simulink model "GUIADO1"  (R2021b)
settings: Solver=VariableStepAuto  StartTime=0.0  StopTime=10.0  RelTol=1e-3
values from neighbouring files (symbols this model uses):
  fp = [t1;t2;t3]    [creacionestructurasborrador.m]    (also in flight_plan.m = [sid,wps,iap]; flight_plan_eval.m = [t1;tabla2;t3]; flight_plan_old.m = [sid,wps,iap]; flight_plan_struct.m = [t1;tabla2;t3])
libraries: simulink x4
settings Model: Creator=patri  LastModifiedBy=verti

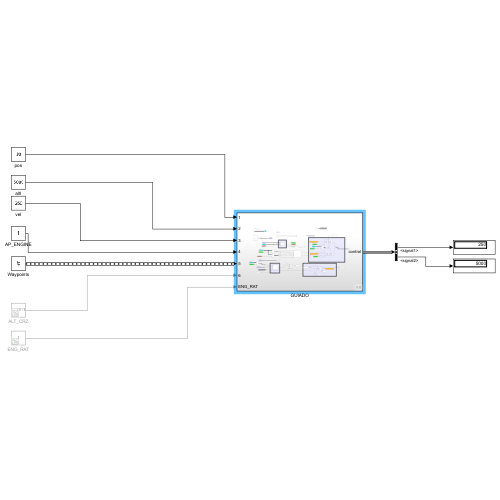
[thumbnail: Simulink's stored preview of the top-level diagram]
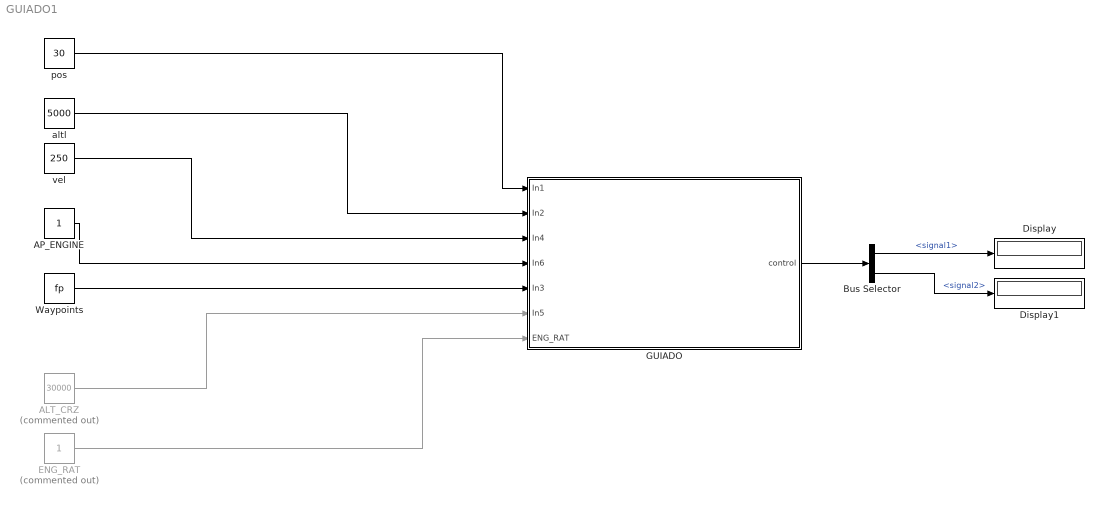
== system GUIADO1 ==
  ALT_CRZ : Constant  Commented=on  Value=30000
  AP_ENGINE : Constant
  Bus Selector : BusSelector  OutputSignals=signal1,signal2
  Display : Display
  Display1 : Display
  ENG_RAT : Constant  Commented=on
  GUIADO : Subsystem
  Waypoints : Constant  RequirementInfo={} %GIDa_b85dfdf9_dbd9_42fc_8c21_ccd8d1c0f83a  Value=fp  OutDataTypeStr=Bus: BUS_FP
  altl : Constant  RequirementInfo={} %GIDa_24b8d891_c115_477c_8ce2_324cbd10ab9b  Value=5000
  pos : Constant  RequirementInfo={} %GIDa_e0c8f14f_9d58_42a1_8d51_6b8f44cf598c  Value=30
  vel : Constant  RequirementInfo={} %GIDa_4ea119f1_ae62_469e_9a59_9854960f9910  Value=250
  wires:
  altl/1 -> GUIADO/2(In2)
  pos/1 -> GUIADO/1(In1)
  vel/1 -> GUIADO/3(In4)
  Waypoints/1 -> GUIADO/5(In3)
  ENG_RAT/1 -> GUIADO/7(ENG_RAT)
  ALT_CRZ/1 -> GUIADO/6(In5)
  AP_ENGINE/1 -> GUIADO/4(In6)
  GUIADO/1(control) -> Bus Selector/1
  Bus Selector/2 -> Display1/1  "<signal2>"
  Bus Selector/1 -> Display/1  "<signal1>"

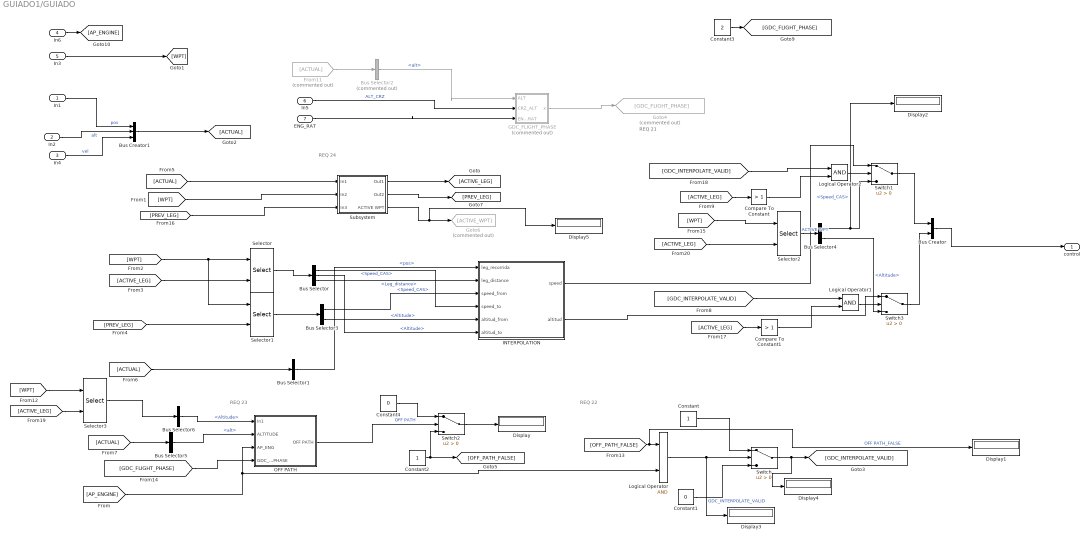
== system GUIADO1/GUIADO ==
  note: REQ 24
  note: REQ 21
  note: REQ 22
  note: REQ 23
  In1 : Inport  RequirementInfo={} %GIDa_c953edaa_2252_4c9d_8426_3d6d548ae88e
  In2 : Inport  RequirementInfo={} %GIDa_547d8447_87e3_4c66_b2f0_2f18738a3143  Port=2
  In4 : Inport  Port=3
  In6 : Inport  Port=4
  In3 : Inport  Port=5
  In5 : Inport  Port=6
  ENG_RAT : Inport  Port=7
  Bus Creator : BusCreator  RequirementInfo={} %GIDa_01f04d6e_35c0_4dde_ad67_30f95352da07  Inputs=2
  Bus Creator1 : BusCreator  RequirementInfo={} %GIDa_002cc265_eead_4a65_9c30_5969614079fc  Inputs=3
  Bus Selector : BusSelector  RequirementInfo={} %GIDa_c4a2b3b9_26f5_4370_8f3c_fb220d56f2b1  OutputSignals=Speed_CAS,Altitude,Leg_distance
  Bus Selector1 : BusSelector  RequirementInfo={} %GIDa_f06f846a_f20a_4ebb_91a5_5d7a160146ce  OutputSignals=pos
  Bus Selector2 : BusSelector  RequirementInfo={} %GIDa_67f18f8f_3d6a_4122_98a0_2b1872e91802  Commented=on  OutputSignals=alt
  Bus Selector3 : BusSelector  RequirementInfo={} %GIDa_3179e8d2_440f_49e3_a760_530bcd082419  OutputSignals=Speed_CAS,Altitude
  Bus Selector4 : BusSelector  OutputSignals=Speed_CAS,Altitude
  Bus Selector5 : BusSelector  OutputSignals=alt
  Bus Selector6 : BusSelector  RequirementInfo={} %GIDa_8bc3223d_0b7f_40fb_a6f5_c44549fe0063  OutputSignals=Altitude
  Compare To Constant : simulink/Logic and Bit Operations/Compare To Constant  relop=>  const=1  OutDataTypeStr=boolean
  Compare To Constant1 : simulink/Logic and Bit Operations/Compare To Constant  relop=>  const=1  OutDataTypeStr=boolean
  Constant : Constant  RequirementInfo={} %GIDa_2498b4de_2ac4_48bd_8c57_f50d97e9c0ba
  Constant1 : Constant  RequirementInfo={} %GIDa_d7690ee0_1221_4b71_bf56_b8fc32b8c303  Value=0
  Constant2 : Constant  RequirementInfo={} %GIDa_5ab9040d_ce11_44b0_aa60_fbd51e1cd284
  Constant3 : Constant  Value=2
  Constant4 : Constant  Value=0
  Display{,1..5} (6 alike) : Display
      Display settings: RequirementInfo={} %GIDa_70cf4f96_cbbf_4ac9_a295_881ac1100427
  From11 : From  RequirementInfo={} %GIDa_ba6d5a2b_274e_4e09_a48e_951a476e8210  Commented=on  GotoTag=ACTUAL
  GDC_FLIGHT_PHASE : Stateflow chart  RequirementInfo={} %GIDa_738fd6ca_d950_41b5_85a8_34e3c94ad36e  Commented=on  TreatAsAtomicUnit=on
  Goto4 : Goto  RequirementInfo={} %GIDa_7a49e31f_81d1_4690_999b_ac34b1e525ce  Commented=on  GotoTag=GDC_FLIGHT_PHASE
  Goto6 : Goto  RequirementInfo={} %GIDa_8f7bf202_a020_4678_839c_04c19c1a886f  Commented=on  GotoTag=ACTIVE_WPT
  INTERPOLATION : MATLAB Function  RequirementInfo={} %GIDa_d69dad2e_6c63_4369_b768_ec321f42f021  TreatAsAtomicUnit=on
  Logical Operator : Logic  RequirementInfo={} %GIDa_5b6a2d32_a21a_44cf_8e21_c6f9ba66fa3f  AllPortsSameDT=off  OutDataTypeStr=boolean
  Logical Operator1 : Logic  RequirementInfo={} %GIDa_0c25b4f0_cec9_4cfd_a32d_1709ca197c58  AllPortsSameDT=off  OutDataTypeStr=boolean
  Logical Operator2 : Logic  RequirementInfo={} %GIDa_21f84cc6_6a89_4154_be44_27295376b10c  AllPortsSameDT=off  OutDataTypeStr=boolean
  OFF PATH : Subsystem  RequirementInfo={} %GIDa_fce4e217_4c17_48f9_b389_237c9766bcea
  Selector : Selector  RequirementInfo={} %GIDa_aa8aed47_c89b_4cd5_946f_b9cf7f706766  InputPortWidth=12  IndexOptions=Index vector (port)  Indices=[1 3]  OutputSizes=1
  Selector1 : Selector  RequirementInfo={} %GIDa_3f3fe1df_2ad1_4bff_9a1e_105282a61a3c  InputPortWidth=12  IndexOptions=Index vector (port)  Indices=[1 3]  OutputSizes=1
  Selector2 : Selector  RequirementInfo={} %GIDa_63b54d3c_663a_435b_9dc1_1443cfa2f20c  InputPortWidth=12  IndexOptions=Index vector (port)  Indices=[1 3]  OutputSizes=1
  Selector3 : Selector  InputPortWidth=12  IndexOptions=Index vector (port)  Indices=[1 3]  OutputSizes=1
  Subsystem : Subsystem  RequirementInfo={} %GIDa_d93d8f36_c3e8_4324_81a1_465d92c3f292
  Switch : Switch  RequirementInfo={} %GIDa_1e34e9e4_1641_447b_8b9c_841ac2d26e67  Criteria=u2 > Threshold
  Switch1 : Switch  RequirementInfo={} %GIDa_27784f20_4fa4_452b_ae6f_1814d084a7da  Criteria=u2 > Threshold
  Switch2 : Switch  RequirementInfo={} %GIDa_46de363e_4d07_48d3_90c2_fbede5ff2297  Criteria=u2 > Threshold
  Switch3 : Switch  RequirementInfo={} %GIDa_d53d12ca_965a_40d8_8672_d8cd2ef96e8e  Criteria=u2 > Threshold
  control : Outport  RequirementInfo={} %GIDa_4dbd6388_d035_474b_bcb7_a1e098248e58
  wires:
  [ACTUAL] -> Bus Selector5/1
  Bus Selector/1 -> INTERPOLATION/4(speed_to)  "<Speed_CAS>"
  Compare To Constant/1 -> Logical Operator2/2
  Constant1/1 -> Switch/3
  Selector1/1 -> Bus Selector3/1
  Switch/1 -> Display4/1, [GDC_INTERPOLATE_VALID]
  Subsystem/2(Out2) -> [PREV_LEG]
  From11/1 -> Bus Selector2/1
  Switch2/1 -> Display/1
  [GDC_FLIGHT_PHASE] -> OFF PATH/4(GDC_FLIGHT_PHASE)
  [ACTUAL] -> Subsystem/1(In1)
  Bus Selector3/1 -> INTERPOLATION/3(speed_from)  "<Speed_CAS>"
  Bus Selector3/2 -> INTERPOLATION/5(altitud_from)  "<Altitude>"
  In2/1 -> Bus Creator1/2  "alt"
  INTERPOLATION/1(speed) -> Switch1/1
  [ACTIVE_LEG] -> Compare To Constant/1
  Compare To Constant1/1 -> Logical Operator1/2
  Logical Operator2/1 -> Switch1/2
  [ACTIVE_LEG] -> Compare To Constant1/1
  Constant2/1 -> Switch2/3, [OFF_PATH_FALSE]
  Switch3/1 -> Bus Creator/2
  [GDC_INTERPOLATE_VALID] -> Logical Operator2/1
  Logical Operator1/1 -> Switch3/2
  [WPT] -> Subsystem/2(In2)
  In3/1 -> [WPT]
  INTERPOLATION/2(altitud) -> Switch3/1
  Bus Creator/1 -> control/1
  Bus Selector/2 -> INTERPOLATION/6(altitud_to)  "<Altitude>"
  Switch1/1 -> Bus Creator/1
  Bus Selector2/1 -> GDC_FLIGHT_PHASE/1(ALT)  "<alt>"
  Constant/1 -> Switch/1
  Logical Operator/1 -> Display3/1, Switch/2  "GDC_INTERPOLATE_VALID"
  Bus Creator1/1 -> [ACTUAL]
  Selector/1 -> Bus Selector/1
  [AP_ENGINE] -> OFF PATH/3(AP_ENG), Logical Operator/2
  [OFF_PATH_FALSE] -> Display1/1, Logical Operator/1  "OFF PATH_FALSE"
  In1/1 -> Bus Creator1/1  "pos"
  [PREV_LEG] -> Subsystem/3(In3)
  [ACTUAL] -> Bus Selector1/1
  Constant4/1 -> Switch2/1
  GDC_FLIGHT_PHASE/1(x) -> Goto4/1
  [WPT] -> Selector1/1, Selector/1
  Subsystem/1(Out1) -> [ACTIVE_LEG]
  OFF PATH/1(OFF PATH) -> Switch2/2  "OFF PATH"
  [GDC_INTERPOLATE_VALID] -> Logical Operator1/1
  [ACTIVE_LEG] -> Selector/2
  In4/1 -> Bus Creator1/3  "vel"
  [ACTIVE_LEG] -> Selector2/2
  [WPT] -> Selector2/1
  Selector2/1 -> Bus Selector4/1  "ACTIVE WPT"
  Bus Selector4/1 -> Display2/1, Switch1/3  "<Speed_CAS>"
  Bus Selector4/2 -> Switch3/3  "<Altitude>"
  [PREV_LEG] -> Selector1/2
  In5/1 -> GDC_FLIGHT_PHASE/2(CRZ_ALT)  "ALT_CRZ"
  ENG_RAT/1 -> GDC_FLIGHT_PHASE/3(ENG_RAT)
  Constant3/1 -> [GDC_FLIGHT_PHASE]
  Bus Selector5/1 -> OFF PATH/2(ALTITUDE)  "<alt>"
  Bus Selector6/1 -> OFF PATH/1(In1)  "<Altitude>"
  [WPT] -> Selector3/1
  Selector3/1 -> Bus Selector6/1
  [ACTIVE_LEG] -> Selector3/2
  In6/1 -> [AP_ENGINE]
  Bus Selector1/1 -> INTERPOLATION/1(leg_recorrida)  "<pos>"
  Bus Selector/3 -> INTERPOLATION/2(leg_distance)  "<Leg_distance>"
  Subsystem/3(ACTIVE WPT) -> Display5/1, Goto6/1

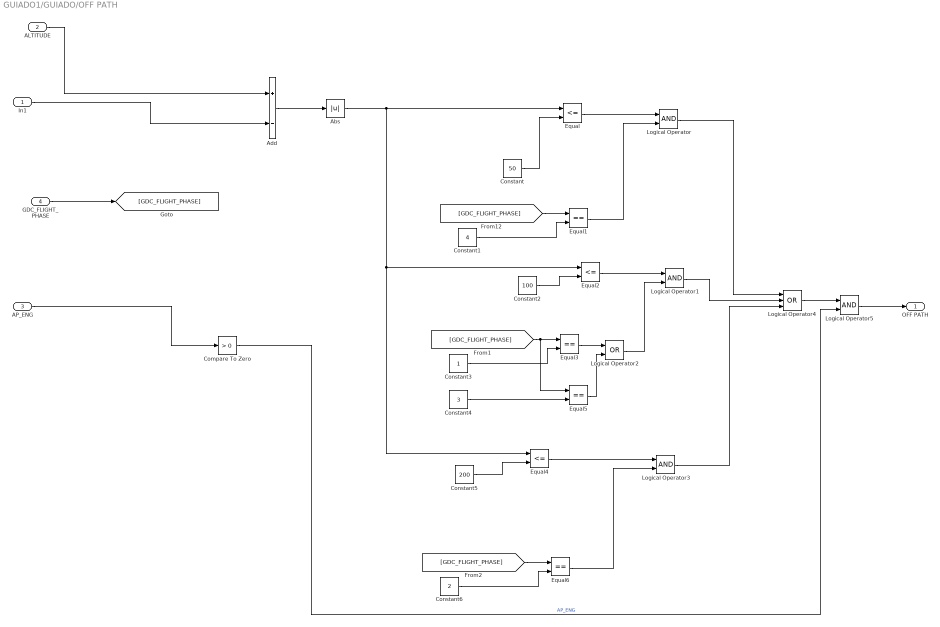
== system GUIADO1/GUIADO/OFF PATH ==
  In1 : Inport  RequirementInfo={} %GIDa_ea188e89_eef4_4315_b4ea_694436859049
  ALTITUDE : Inport  RequirementInfo={} %GIDa_cec92ccd_50af_48ce_99e0_e78f87b5a5dd  Port=2
  AP_ENG : Inport  RequirementInfo={} %GIDa_b5a9fb80_9e70_4b36_a3d4_181a89380a09  Port=3
  GDC_FLIGHT_PHASE : Inport  RequirementInfo={} %GIDa_449a8b27_a283_4b51_85f1_d3db49c09d81  Port=4
  Abs : Abs  RequirementInfo={} %GIDa_db76a9bc_fd40_41b7_b4e9_c8f1fa3f6419
  Add : Sum  RequirementInfo={} %GIDa_1eb463e1_2c0f_4155_9caf_ebd713becfc9  Inputs=+-
  Compare To Zero : simulink/Logic and Bit Operations/Compare To Zero  RequirementInfo={} %GIDa_de6d2e43_5074_4e60_86a5_29e173b01aeb  relop=>  OutDataTypeStr=boolean
  Constant : Constant  RequirementInfo={} %GIDa_50edc1c4_4358_4970_abca_b0e9409f851a  Value=50
  Constant1 : Constant  RequirementInfo={} %GIDa_ee39c8f9_9d82_4b7c_b7b4_7766ecc2abfe  Value=4
  Constant2 : Constant  RequirementInfo={} %GIDa_fa64b539_4baf_4742_984f_2a1e30e52f84  Value=100
  Constant3 : Constant  RequirementInfo={} %GIDa_b30783bd_8107_4173_8871_ce95e60f06e5
  Constant4 : Constant  RequirementInfo={} %GIDa_62456426_7c96_48d7_b64a_6a8d71b153fa  Value=3
  Constant5 : Constant  RequirementInfo={} %GIDa_6ce19b5c_559d_4c88_b743_76247ddbb29b  Value=200
  Constant6 : Constant  RequirementInfo={} %GIDa_176fc83c_97bb_40dd_8d0a_c2bcedeeb068  Value=2
  Equal : RelationalOperator  RequirementInfo={} %GIDa_461bf3d0_5128_4580_83eb_d11cda6f1f54  Operator=<=  OutDataTypeStr=boolean  RndMeth=Simplest
  Equal1 : RelationalOperator  RequirementInfo={} %GIDa_fb95551d_c38f_4b25_a200_648df0e3a261  Operator===  OutDataTypeStr=boolean  RndMeth=Simplest
  Equal2 : RelationalOperator  RequirementInfo={} %GIDa_07670def_aa68_4caa_b5d3_7fed440a0cb2  Operator=<=  OutDataTypeStr=boolean  RndMeth=Simplest
  Equal3 : RelationalOperator  RequirementInfo={} %GIDa_ceb44fc0_0920_4a7b_ba38_e15afd348e9c  Operator===  OutDataTypeStr=boolean  RndMeth=Simplest
  Equal4 : RelationalOperator  RequirementInfo={} %GIDa_b1d64c76_31ce_47f0_b5ac_a43420f1547c  Operator=<=  OutDataTypeStr=boolean  RndMeth=Simplest
  Equal5 : RelationalOperator  RequirementInfo={} %GIDa_2958bcab_fb85_461e_97e2_a6dac5bfcaec  Operator===  OutDataTypeStr=boolean  RndMeth=Simplest
  Equal6 : RelationalOperator  RequirementInfo={} %GIDa_58d89293_8496_455d_9e80_32ec11f8f5c1  Operator===  OutDataTypeStr=boolean  RndMeth=Simplest
  Logical Operator : Logic  RequirementInfo={} %GIDa_cea7d4b5_5f50_4197_98d6_c45754679a30  AllPortsSameDT=off  OutDataTypeStr=boolean
  Logical Operator1 : Logic  RequirementInfo={} %GIDa_f384c015_dcc1_4c97_bf18_ececb565dac7  AllPortsSameDT=off  OutDataTypeStr=boolean
  Logical Operator2 : Logic  RequirementInfo={} %GIDa_d6ad186f_4603_4263_8868_992f6354fea7  Operator=OR  AllPortsSameDT=off  OutDataTypeStr=boolean
  Logical Operator3 : Logic  RequirementInfo={} %GIDa_7655793f_75d5_490d_973e_06ad41c3d157  AllPortsSameDT=off  OutDataTypeStr=boolean
  Logical Operator4 : Logic  RequirementInfo={} %GIDa_9854a055_86ef_4427_9c40_3c0f9a0ce9c4  Operator=OR  Inputs=3  AllPortsSameDT=off  OutDataTypeStr=boolean
  Logical Operator5 : Logic  RequirementInfo={} %GIDa_f127f70b_32ec_43f5_ae91_9e69a0f60159  AllPortsSameDT=off  OutDataTypeStr=boolean
  OFF PATH : Outport  RequirementInfo={} %GIDa_2c7fbac8_b281_4014_84d4_14cf9235134e
  wires:
  AP_ENG/1 -> Compare To Zero/1
  Compare To Zero/1 -> Logical Operator5/2  "AP_ENG"
  ALTITUDE/1 -> Add/1
  Add/1 -> Abs/1
  Constant/1 -> Equal/2
  Abs/1 -> Equal4/1, Equal2/1, Equal/1
  [GDC_FLIGHT_PHASE] -> Equal1/1
  Constant1/1 -> Equal1/2
  Equal1/1 -> Logical Operator/2
  Equal/1 -> Logical Operator/1
  Constant2/1 -> Equal2/2
  Constant3/1 -> Equal3/2
  [GDC_FLIGHT_PHASE] -> Equal5/1, Equal3/1
  Equal2/1 -> Logical Operator1/1
  Equal3/1 -> Logical Operator2/1
  Constant4/1 -> Equal5/2
  Equal5/1 -> Logical Operator2/2
  Logical Operator2/1 -> Logical Operator1/2
  Constant5/1 -> Equal4/2
  Constant6/1 -> Equal6/2
  [GDC_FLIGHT_PHASE] -> Equal6/1
  Equal6/1 -> Logical Operator3/2
  Equal4/1 -> Logical Operator3/1
  Logical Operator/1 -> Logical Operator4/1
  Logical Operator1/1 -> Logical Operator4/2
  Logical Operator3/1 -> Logical Operator4/3
  Logical Operator4/1 -> Logical Operator5/1
  In1/1 -> Add/2
  Logical Operator5/1 -> OFF PATH/1
  GDC_FLIGHT_PHASE/1 -> [GDC_FLIGHT_PHASE]

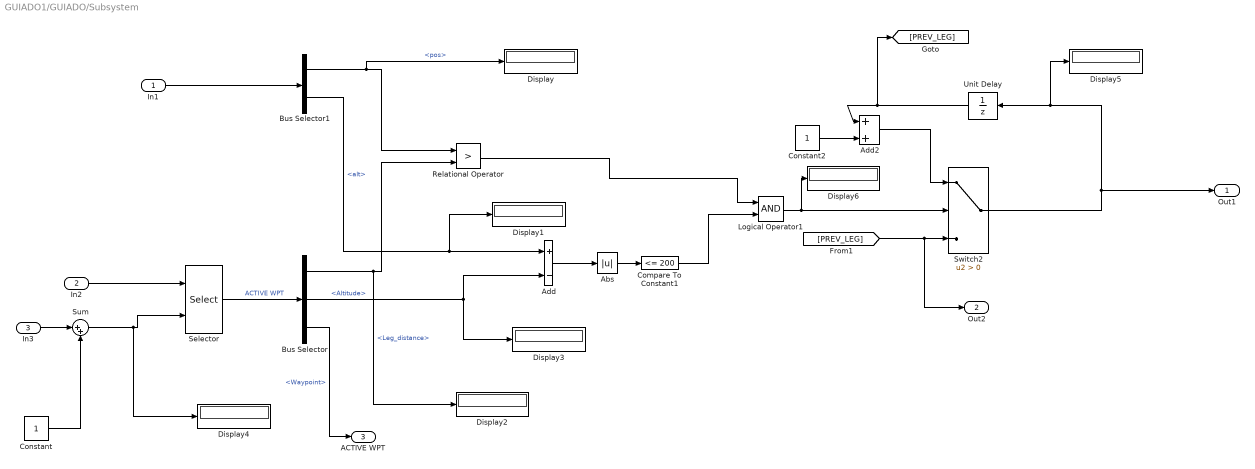
== system GUIADO1/GUIADO/Subsystem ==
  In1 : Inport  RequirementInfo={} %GIDa_0131d32b_efee_4ea4_ac79_6c0467cb0f93
  In2 : Inport  RequirementInfo={} %GIDa_9332eabb_72a9_49df_8cfa_42eb4af22996  Port=2
  In3 : Inport  RequirementInfo={} %GIDa_dcaabb5c_a970_4c12_84e6_593f38f6e7eb  Port=3
  Abs : Abs  RequirementInfo={} %GIDa_2ae6489e_018f_40d7_8bb4_c77ff0e16f9a
  Add : Sum  RequirementInfo={} %GIDa_7a86c0f9_7540_49ad_840d_54a1c2d08e41  Inputs=+-
  Add2 : Sum  RequirementInfo={} %GIDa_69bf13d4_be9d_421e_9007_68151da1e8fe
  Bus Selector : BusSelector  RequirementInfo={} %GIDa_38129ef7_1831_4e83_9593_e617cd59c72a  OutputSignals=Leg_distance,Altitude,Waypoint
  Bus Selector1 : BusSelector  RequirementInfo={} %GIDa_02b0c3c9_c6c4_4e49_9650_2eb0e6fcee0e  OutputSignals=pos,alt
  Compare To Constant1 : simulink/Logic and Bit Operations/Compare To Constant  RequirementInfo={} %GIDa_29eeb14b_64e1_47ad_a8b8_57d14cc1056b  relop=<=  const=200  OutDataTypeStr=boolean
  Constant : Constant  RequirementInfo={} %GIDa_8c597851_388c_4980_a07b_e0390fd17eb0
  Constant2 : Constant  RequirementInfo={} %GIDa_09d14399_5cb7_4ffd_9a54_cc5e11d9388d
  Display{,1..6} (7 alike) : Display
      Display settings: RequirementInfo={} %GIDa_699eee58_7c59_4805_8ad2_3d54e1a4e210
      Display1 settings: RequirementInfo={} %GIDa_a74b27ed_38af_4b0c_8e4e_74dbd8697a6b
      Display2 settings: RequirementInfo={} %GIDa_92650422_1419_4ef5_8e7f_eb2107227185
      Display3 settings: RequirementInfo={} %GIDa_8ba27ae7_890a_4709_96d0_b73deccccb71
      Display4 settings: RequirementInfo={} %GIDa_5fb75b9b_3fad_4f3d_8fd4_d5d146326274
  Logical Operator1 : Logic  RequirementInfo={} %GIDa_892ee212_3d47_43e5_b94b_21bb92133837  AllPortsSameDT=off  OutDataTypeStr=boolean
  Relational Operator : RelationalOperator  RequirementInfo={} %GIDa_791e8e3d_0bb6_41cc_b451_066d914e6f49  Operator=>  OutDataTypeStr=boolean  RndMeth=Simplest
  Selector : Selector  RequirementInfo={} %GIDa_c6254e5f_2d4b_4f8b_a442_8bcc3cde2ca2  InputPortWidth=12  IndexOptions=Index vector (port)  Indices=[1 3]  OutputSizes=1
  Sum : Sum  RequirementInfo={} %GIDa_ec62c27e_9ee3_4b0a_b964_4e78006d0ed7  Inputs=|++
  Switch2 : Switch  RequirementInfo={} %GIDa_fc591049_3db6_4272_a4c0_26dfbcb57961  Criteria=u2 > Threshold
  Unit Delay : UnitDelay  RequirementInfo={} %GIDa_2b3ed8d6_cf04_4ce4_aa86_d5ea7e51b5cf  InitialCondition=1  SampleTime=-1  HasFrameUpgradeWarning=on
  Out1 : Outport  RequirementInfo={} %GIDa_e9e5d1ca_d56d_4e46_83b3_5997bde3cb88
  Out2 : Outport  RequirementInfo={} %GIDa_ae771310_bfb2_4d29_8529_65097305e090  Port=2
  ACTIVE WPT : Outport  RequirementInfo={} %GIDa_7d6f1c26_7e2a_42d4_8a20_168f26657803  Port=3
  wires:
  Add/1 -> Abs/1
  Add2/1 -> Switch2/1
  Unit Delay/1 -> Add2/1, [PREV_LEG]
  Constant2/1 -> Add2/2
  Bus Selector1/2 -> Display1/1, Add/1  "<alt>"
  Relational Operator/1 -> Logical Operator1/1
  Bus Selector1/1 -> Display/1, Relational Operator/1  "<pos>"
  Logical Operator1/1 -> Display6/1, Switch2/2
  [PREV_LEG] -> Out2/1, Switch2/3
  Selector/1 -> Bus Selector/1  "ACTIVE WPT"
  Bus Selector/1 -> Display2/1, Relational Operator/2  "<Leg_distance>"
  Compare To Constant1/1 -> Logical Operator1/2
  Abs/1 -> Compare To Constant1/1
  Bus Selector/2 -> Add/2, Display3/1  "<Altitude>"
  In2/1 -> Selector/1
  In1/1 -> Bus Selector1/1
  Switch2/1 -> Out1/1, Display5/1, Unit Delay/1
  Constant/1 -> Sum/2
  Bus Selector/3 -> ACTIVE WPT/1  "<Waypoint>"
  In3/1 -> Sum/1
  Sum/1 -> Display4/1, Selector/2

== stateflow chart GUIADO1/GUIADO/GDC_FLIGHT_PHASE ==
  state CLIMB
    entry:
    x = 1;
  state CRUISE
    entry:
    x = 2;
  state DESCEND
    entry:
    x = 3;
  state APPROACH
    entry:
    x=4;
  (default) -> CLIMB
  DESCEND -> APPROACH : [ALT<2000]
  CLIMB -> CRUISE : [ALT>=CRZ_ALT]
  CRUISE -> DESCEND [order 2] : [(ALT<CRZ_ALT) & (ENG_RAT==IDLE)]
  CRUISE -> CLIMB [order 1] : [ALT<CRZ_ALT & (ENG_RAT==MTO | ENG_RAT==MCT | ENG_RAT==CLB)]
  data: ALT input; x output; CLB constant double =2; MTO constant double =4; CRZ_ALT input; IDLE constant double =1; MCT constant double =3; ENG_RAT input

== matlab function GUIADO1/GUIADO/INTERPOLATION ==
  data: leg_recorrida input; leg_distance input; speed_from input; speed_to input; altitud_from input; speed output; altitud_to input; altitud output
function [speed,altitud] = mapeo(leg_recorrida,leg_distance,speed_from,speed_to,altitud_from,altitud_to)

speed = (leg_recorrida) .* (speed_to - speed_from) ./ (leg_distance) + speed_from;

altitud = (leg_recorrida) .* (altitud_to - altitud_from) ./ (leg_distance) + altitud_from;

end

% function [vel,alt]  = interpolate(actWPTvel, actWPTalt, prevWPTvel, prevWPTalt, Actual_pointvel, Actual_pointalt)
% 
% vel = prevWPTvel + ((actWPTvel-prevWPTvel)/(actWPTalt-prevWPTalt))*(Actual_pointvel);
% 
% alt = prevWPTvel + ((actWPTvel-prevWPTvel)/(actWPTalt-prevWPTalt))*(Actual_pointvel);
